simulink model "simulation"  (R2014a)
settings: Solver=ode45  StartTime=0.0  StopTime=180  RelTol=1e-3
libraries: simulink x1
settings Model: Creator=pk  LastModifiedBy=saura_000
settings DataIOCC: SignalLoggingSaveFormat=ModelDataLogs
settings OptimizationCC: InitFltsAndDblsToZero=on
settings DebuggingCC: SaveWithParameterizedLinksMsg=none  UnderspecifiedInitializationDetection=Classic  SignalResolutionControl=TryResolveAllWithWarning  MultiTaskDSMMsg=warning  MultiTaskCondExecSysMsg=none
settings RTWCC: IncludeERTFirstTime=on
settings GRTTargetCC: TargetFcnLib=ansi_tfl_tmw.mat  CombineOutputUpdateFcns=off  GRTInterface=on

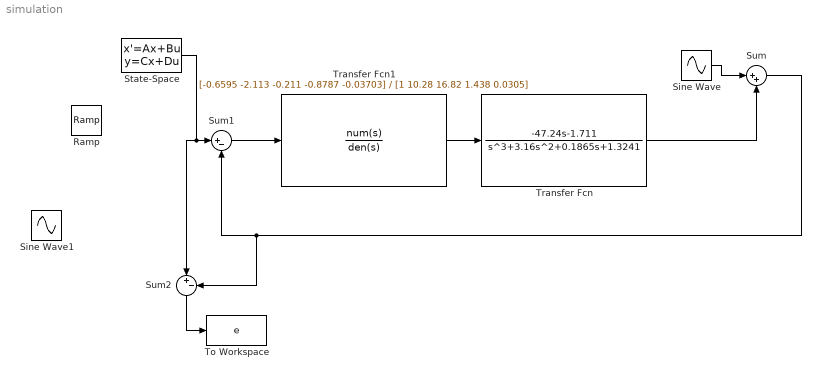
== system simulation ==
  Ramp : simulink/Sources/Ramp  slope=1  start=0  X0=0
  Sine Wave : Sin  SampleTime=0
  Sine Wave1 : Sin  Phase=1.57  SampleTime=0
  State-Space : StateSpace  A=-2  D=0  X0=10
  Sum : Sum  Inputs=|++
  Sum1 : Sum  Inputs=|+-
  Sum2 : Sum  Inputs=|+-
  To Workspace : ToWorkspace  VariableName=e  SaveFormat=Structure With Time  SampleTime=0.01
  Transfer Fcn : TransferFcn  Numerator=[-47.24 -1.711]  Denominator=[1 3.16 0.1865 1.3241]
  Transfer Fcn1 : TransferFcn  Numerator=[-0.6595 -2.113 -0.211 -0.8787 -0.03703]  Denominator=[1 10.28 16.82 1.438 0.0305]
  wires:
  Transfer Fcn/1 -> Sum/2
  Sine Wave/1 -> Sum/1
  Sum/1 -> Sum1/2, Sum2/2
  State-Space/1 -> Sum2/1, Sum1/1
  Sum2/1 -> To Workspace/1
  Transfer Fcn1/1 -> Transfer Fcn/1
  Sum1/1 -> Transfer Fcn1/1
